simulink model "TCAF_WHOLESIM"  (R2022a)
settings: Solver=ode4  StartTime=0.0  StopTime=150  FixedStep=0.01  RelTol=1e-3  EnableMultiTasking=on
PreLoadFcn:
  | listing = dir;
  | if (contains([listing .name], 'TPF')) && (contains([listing .name], 'MAP'))
  |     addpath('./TCAF', './TRN', './FTG', './DYN', './FLCC', './GPS', './RALT', './INS', './MAP');
  | elseif (contains([listing .name], 'TCAF_WHOLESIM.slx'))
  |     addpath('./TCAF', './TRN', './FTG', '../DYN', '../FLCC', '../GPS', '../RALT', '../INS', '../MAP');
  | else
  | 
  | end
  | addpath('C:\Users\ASCL\Documents\GitHub\DTNS\MAP\MAP_DB');
  | 
  | load('BUS_STRUCTURE_DYN.mat');
  | load('BUS_STRUCTURE_FLCC.mat');
  | load('BUS_STRUCTURE_RALT.mat');
  | load('BUS_STRUCTURE_INS.mat');
  | load('BUS_STRUCTURE_GPS.mat');
  | load('BusStructureTRN.mat');
  | load('BusStructureWTPG.mat');
  | load('BusStructureDTF.mat');
  | load('BusStructureGCAWS.mat');
  | FTG_initState;
InitFcn:
  | listing = dir;
  | if (contains([listing .name], 'TPF')) && (contains([listing .name], 'MAP'))
  |     addpath('./TCAF', './TRN', './FTG', './DYN', './FLCC', './GPS', './RALT', './INS', './MAP');
  | elseif (contains([listing .name], 'TCAF_WHOLESIM.slx'))
  |     addpath('./TCAF', './TRN', './FTG', '../DYN', '../FLCC', '../GPS', '../RALT', '../INS', '../MAP');
  | else
  | 
  | end
  | 
  | load('BUS_STRUCTURE_DYN.mat');
  | load('BUS_STRUCTURE_FLCC.mat');
  | load('BUS_STRUCTURE_RALT.mat');
  | load('BUS_STRUCTURE_INS.mat');
  | load('BUS_STRUCTURE_GPS.mat');
  | load('BusStructureTRN.mat');
  | load('BusStructureWTPG.mat');
  | load('BusStructureDTF.mat');
  | load('BusStructureGCAWS.mat');
  | FTG_initState;
  | 
  | clear 'logsout'
libraries: aerolibconvert2 x14, simulink_extras x5
(part 1 of 2)
settings Model: PacingRate=3  Creator=ASCL  LastModifiedBy=ASCL
settings SolverCC: PositivePriorityOrder=on  AutoInsertRateTranBlk=on
settings DataIOCC: ExternalInput=FTGScenario.getElement('IN_STICK'), [], [], FTGScenario.getElement('IN_FLIGHT_CMD'), []  LoadExternalInput=on  SaveOutput=off  DSMLogging=off  ReturnWorkspaceOutputs=off
settings OptimizationCC: BlockReduction=off  DefaultParameterBehavior=Inlined  UseDivisionForNetSlopeComputation=on  GainParamInheritBuiltInType=on  UseFloatMulNetSlope=on  ExpressionFolding=off  PassReuseOutputArgsAs=Individual arguments  ZeroExternalMemoryAtStartup=off  ZeroInternalMemoryAtStartup=off  EfficientFloat2IntCast=on  LifeSpan=inf  OptimizeBlockOrder=speed  DifferentSizesBufferReuse=on  EfficientTunableParamExpr=on
settings DebuggingCC: SignalInfNanChecking=warning  ReadBeforeWriteMsg=EnableAllAsError  WriteAfterWriteMsg=EnableAllAsError  WriteAfterReadMsg=EnableAllAsError  IntegerOverflowMsg=error  ParameterTunabilityLossMsg=error  UniqueDataStoreMsg=error  AssertControl=DisableAll  NonBusSignalsTreatedAsBus=error  SFInvalidInputDataAccessInChartInitDiag=error  SFTransitionOutsideNaturalParentDiag=error  SFUnreachableExecutionPathDiag=error  SFUndirectedBroadcastEventsDiag=error  IntegerSaturationMsg=error
settings HardwareCC: ProdBitPerPointer=32  ProdBitPerSizeT=32  ProdBitPerPtrDiffT=32  ProdLargestAtomicInteger=Long  ProdLargestAtomicFloat=Double  ProdEndianess=BigEndian  ProdWordSize=32  ProdLongLongMode=on  ProdHWDeviceType=Freescale->MPC83xx
settings ModelReferenceCC: ModelReferenceNumInstancesAllowed=Single
settings SFSimCC: SimCustomHeaderCode="#include \"MAP.h\""  SimUserSources=MAP.c  SimUserLibraries=WS2_32.LIB  CompileTimeRecursionLimit=0  EnableRuntimeRecursion=off  MATLABDynamicMemAlloc=off  CustomCodeGlobalsAsFunctionIO=on
settings RTWCC: SystemTargetFile=ert.tlc  TemplateMakefile=ert_default_tmf  GenerateReport=on  RTWUseSimCustomCode=on  CustomHeaderCode="#include \"MAP.h\""  CustomSource=MAP.c  CustomLibrary=WS2_32.LIB  BuildConfiguration=Faster Runs  IncludeHyperlinkInReport=on  LaunchReport=on  GenerateTraceInfo=on  GenerateTraceReport=on  GenerateTraceReportSl=on  GenerateTraceReportSf=on  GenerateTraceReportEml=on
settings CodeAppCC: ForceParamTrailComments=on  IgnoreCustomStorageClasses=off  OperatorAnnotations=on  SimulinkDataObjDesc=on  SFDataObjDesc=on  MATLABFcnDesc=on  InsertBlockDesc=on  StateflowObjectComments=on  MATLABSourceComments=on  EnableCustomComments=on  InlinedPrmAccess=Macros  ReqsInCode=on
settings ERTTargetCC: TargetLangStandard=C99 (ISO)  UtilityFuncGeneration=Shared location  GenerateSampleERTMain=on  IncludeMdlTerminateFcn=off  CombineSignalStateStructs=on  SuppressErrorStatus=on  SupportAbsoluteTime=off  SupportNonFinite=off  SupportComplex=off  ParenthesesLevel=Standards  CastingMode=Standards  GenerateSharedConstants=off  InlinedParameterPlacement=NonHierarchical  ERTCustomFileTemplate=example_file_process.tlc  RateTransitionBlockCode=Function  PreserveIfCondition=on  ConvertIfToSwitch=off  EnableSignedLeftShifts=off  EnableSignedRightShifts=off

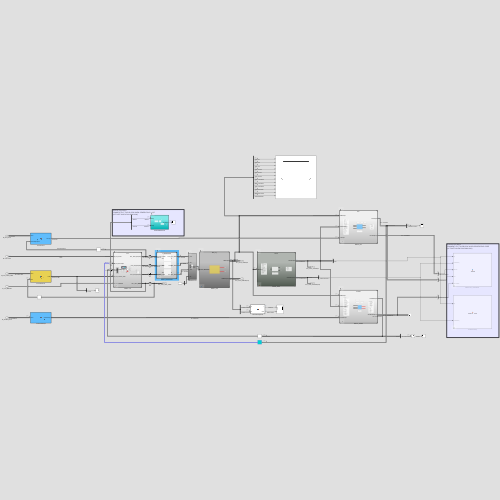
[thumbnail: Simulink's stored preview of the top-level diagram]
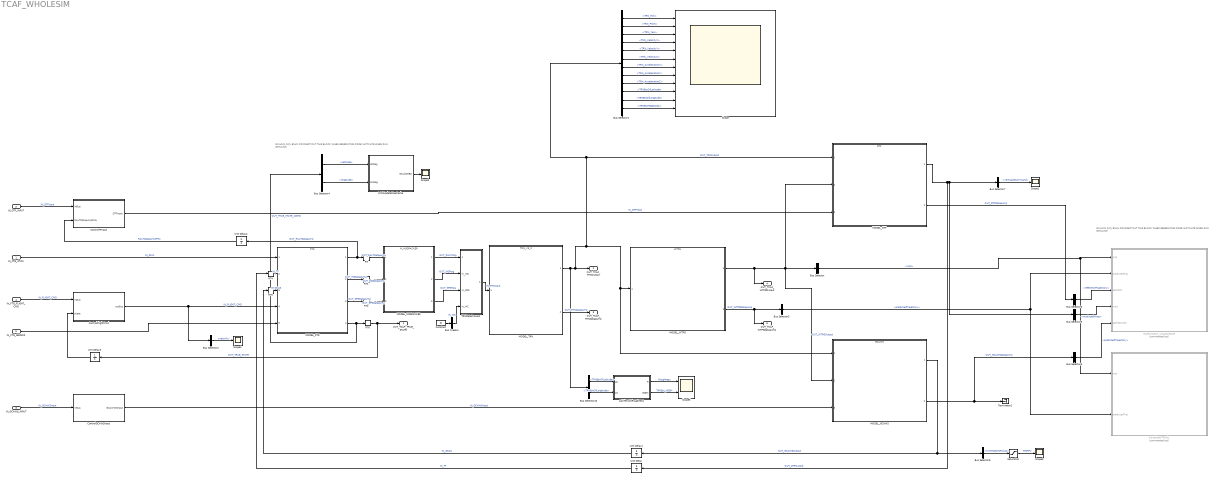
== system TCAF_WHOLESIM ==
  note: Simulink Only Block
      | COMMENT OUT THIS BLOCK WHEN GENERATING CODE
      | (ACTIVATE WHEN RUN SIMULINK)
  note: Simulink Only Block
      | COMMENT OUT THIS BLOCK WHEN GENERATING CODE
      | (ACTIVATE WHEN RUN SIMULINK)
  IN_FTG_STICK : Inport  OutDataTypeStr=Bus: BUS_FLCC_STICK  BusOutputAsStruct=on
  IN_DTF_INPUT : Inport  Port=2  OutDataTypeStr=Bus: DTFInput  BusOutputAsStruct=on
  IN_GCAWS_INPUT : Inport  Port=3  OutDataTypeStr=Bus: GCAWSInput  BusOutputAsStruct=on
  IN_FTG_FLIGHT_CMD : Inport  Port=4  OutDataTypeStr=Bus: BUS_FLCC_FLIGHT_CMD  Interpolate=off  BusOutputAsStruct=on
  IN_FTG_SENSOR : Inport  Port=5  OutDataTypeStr=Bus: BUS_SENSOR_ALL_INPUTSTATUS  BusOutputAsStruct=on
  Bus Creator : BusCreator  Inputs=1  OutDataTypeStr=Bus: TRN_MC  NonVirtualBus=on
      settings: InheritFromInputs=off
  Bus Selector : BusSelector  OutputSignals=wtp
  Bus Selector1 : BusSelector  OutputSignals=TRN_Roll,TRN_Pitch,TRN_Yaw,TRN_VelocityX,TRN_VelocityY,TRN_VelocityZ,TRN_AccelerationX,TRN_AccelerationY,TRN_AccelerationZ,TRNEstOfLatitude,TRNEstOfLongitude,TRNEstHeightAGL
  Bus Selector10 : BusSelector  OutputSignals=TRNEstOfLatitude,TRNEstOfLongitude
  Bus Selector2 : BusSelector  OutputSignals=nextAlt
  Bus Selector3 : BusSelector  OutputSignals=predictedTrajectory
  Bus Selector4 : BusSelector  OutputSignals=latitude,longitude
  Bus Selector5 : BusSelector  OutputSignals=predictedTrajectory
  Bus Selector6 : BusSelector  OutputSignals=referenceTrajectory
  Bus Selector7 : BusSelector  OutputSignals=verticalGCommand
  Bus Selector8 : BusSelector  OutputSignals=timeToGoToPullUp
  Bus Selector9 : BusSelector  OutputSignals=msdUsedWrap
  Constant : Constant  Value=0  OutDataTypeStr=boolean
  ControlFlightCmd : MATLAB Function  TreatAsAtomicUnit=on
  ControlGCAWSInput : MATLAB Function  TreatAsAtomicUnit=on
  ControlTFInput : MATLAB Function  TreatAsAtomicUnit=on
  InitNUpdateMapCache : Subsystem  TreatAsAtomicUnit=on  ScheduleAs=Periodic partition  PartitionName=InitNUpdateMapCache  SystemSampleTime=0.01
  MATFunction_VisualizeWCP : MATLAB Function  Commented=on  TreatAsAtomicUnit=on
  MODEL_DTF : ModelReference  ModelNameDialog=DTF.slx  SimulationMode=Normal  ScheduleRates=on  ScheduleRatesWith=Schedule Editor  ModelReferenceVersion=1.433
  MODEL_FTG : ModelReference  ModelNameDialog=FTG.slx  SimulationMode=Normal  ScheduleRates=on  ScheduleRatesWith=Schedule Editor  ModelReferenceVersion=1.514
  MODEL_GCAWS : ModelReference  ModelNameDialog=GCAWS.slx  SimulationMode=Normal  ScheduleRates=on  ScheduleRatesWith=Schedule Editor  ModelReferenceVersion=1.778
  MODEL_MSGPACKER : ModelReference  ModelNameDialog=M_MSGPACKER.slx  SimulationMode=Normal  ScheduleRates=on  ScheduleRatesWith=Schedule Editor  ModelReferenceVersion=1.311
  MODEL_TRN : ModelReference  ModelNameDialog=TRN_V3_2.slx  SimulationMode=Normal  ScheduleRates=on  ScheduleRatesWith=Schedule Editor  CachedPortDiscreteRates=[0.04]  ModelReferenceVersion=2.345
  MODEL_WTPG : ModelReference  ModelNameDialog=WTPG.slx  SimulationMode=Normal  ScheduleRates=on  ScheduleRatesWith=Schedule Editor  ModelReferenceVersion=1.378
  RT{,1..2,4..5} (5 alike) : RateTransition
  RT6 : RateTransition  OutPortSampleTime=0.04
  Saturation : Saturate  UpperLimit=5.0  LowerLimit=0.0
  Scope : Scope  NumInputPorts=12
  Scope{1..4} (4 alike) : Scope
  Scope5 : Scope  NumInputPorts=2
  TRNDataProcess : Subsystem  TreatAsAtomicUnit=on  ScheduleAs=Periodic partition  PartitionName=TRNDataProcess  SystemSampleTime=0.04
  Terminator2 : Terminator
  Unit Delay{,1..3} (4 alike) : UnitDelay  SampleTime=-1  HasFrameUpgradeWarning=on
  VisualizeWTPOnly : MATLAB Function  Commented=on  TreatAsAtomicUnit=on
  calcTerrainRoughness : MATLAB Function  TreatAsAtomicUnit=on
  OUT_TCAF_TRUE_STATE : Outport  OutDataTypeStr=Bus: BUS_DYN_STATE  BusOutputAsStruct=on
  OUT_TCAF_TRNOutput : Outport  Port=2  OutDataTypeStr=Bus: TRNOutput  BusOutputAsStruct=on
  OUT_TCAF_TRNDatapump : Outport  Port=3  OutDataTypeStr=Bus: TRNDatapump
  OUT_TCAF_WTPGOutput : Outport  Port=4  OutDataTypeStr=Bus: WTPGOutput
  OUT_TCAF_WTPGDatapump : Outport  Port=5  OutDataTypeStr=Bus: WTPGDatapump
  wires:
  Bus Selector7/1 -> Scope1/1  "<verticalGCommand>"
  Bus Selector6/1 -> MATFunction_VisualizeWCP/3(pathDTF)  "<referenceTrajectory>"
  Bus Selector1/4 -> Scope/4  "<TRN_VelocityX>"
  MODEL_DTF/2 -> Bus Selector6/1  "OUT_DTFDatapump"
  Bus Creator/1 -> TRNDataProcess/4(In_MC)  "IN_MC"
  Bus Selector5/1 -> MATFunction_VisualizeWCP/5(pathGCAWS)  "<predictedTrajectory>"
  Bus Selector1/5 -> Scope/5  "<TRN_VelocityY>"
  Bus Selector1/7 -> Scope/7  "<TRN_AccelerationX>"
  Bus Selector1/8 -> Scope/8  "<TRN_AccelerationY>"
  MODEL_WTPG/1 -> OUT_TCAF_WTPGOutput/1, MODEL_GCAWS/2, MODEL_DTF/2, Bus Selector/1  "OUT_WTPGOutput"
  Bus Selector1/9 -> Scope/9  "<TRN_AccelerationZ>"
  Bus Selector1/12 -> Scope/12  "<TRNEstHeightAGL>"
  Bus Selector1/11 -> Scope/11  "<TRNEstOfLongitude>"
  MODEL_FTG/3 -> RT2/1  "OUT_GPSDatapump"
  MODEL_WTPG/2 -> OUT_TCAF_WTPGDatapump/1, Bus Selector3/1  "OUT_WTPGDatapump"
  Bus Selector1/3 -> Scope/3  "<TRN_Yaw>"
  MODEL_GCAWS/2 -> Bus Selector5/1, Terminator2/1  "OUT_GCAWSDatapump"
  Bus Selector1/10 -> Scope/10  "<TRNEstOfLatitude>"
  MODEL_TRN/2 -> OUT_TCAF_TRNDatapump/1  "OUT_TRNDatapump"
  MODEL_GCAWS/1 -> Unit Delay1/1, Bus Selector8/1  "OUT_GCAWSOutput"
  Bus Selector1/6 -> Scope/6  "<TRN_VelocityZ>"
  Bus Selector3/1 -> VisualizeWTPOnly/2(predictedTraj), MATFunction_VisualizeWCP/2(predictedTraj)  "<predictedTrajectory>"
  Constant/1 -> Bus Creator/1
  IN_GCAWS_INPUT/1 -> ControlGCAWSInput/1(inBus)  "IN_GCAWSInput"
  IN_FTG_FLIGHT_CMD/1 -> ControlFlightCmd/1(inBus)  "IN_FLIGHT_CMD"
  RT6/1 -> Unit Delay3/1, OUT_TCAF_TRUE_STATE/1  "OUT_TRUE_STATE"
  Bus Selector4/2 -> InitNUpdateMapCache/2(lonDeg)  "<longitude>"
  MODEL_FTG/2 -> RT1/1  "OUT_INSDatapump"
  Unit Delay1/1 -> RT5/1  "IN_GCAS"
  Unit Delay/1 -> RT4/1  "IN_TF"
  MODEL_FTG/1 -> RT/1, Unit Delay2/1  "OUT_RALTDatapump"
  Bus Selector/1 -> VisualizeWTPOnly/1(wtp), MATFunction_VisualizeWCP/1(wtp)  "<wtp>"
  Bus Selector1/1 -> Scope/1  "<TRN_Roll>"
  IN_FTG_STICK/1 -> MODEL_FTG/1  "IN_Stick"
  MODEL_DTF/1 -> Bus Selector9/1, Bus Selector7/1, Unit Delay/1  "OUT_DTFOutput"
  Bus Selector1/2 -> Scope/2  "<TRN_Pitch>"
  Bus Selector8/1 -> Saturation/1  "<timeToGoToPullUp>"
  Saturation/1 -> Scope3/1  "TTGTPU"
  ControlFlightCmd/1(outBus) -> Bus Selector2/1, MODEL_FTG/4  "IN_FLIGHT_CMD"
  IN_DTF_INPUT/1 -> ControlTFInput/1(inBus)  "IN_DTFInput"
  MODEL_MSGPACKER/3 -> TRNDataProcess/3(In_GPS)  "OUT_GPSMsg"
  MODEL_MSGPACKER/1 -> TRNDataProcess/1(In_RALT)  "OUT_RALTMsg"
  MODEL_MSGPACKER/2 -> TRNDataProcess/2(In_INS)  "OUT_INSMsg"
  InitNUpdateMapCache/1(resultDTED) -> Scope2/1
  IN_FTG_SENSOR/1 -> MODEL_FTG/5
  ControlTFInput/1(DTFInput) -> MODEL_DTF/3  "IN_DTFInput"
  Unit Delay2/1 -> ControlTFInput/2(RALTDatapumpPrev)  "RALTDatapumpPrev"
  Bus Selector2/1 -> Scope4/1  "<nextAlt>"
  ControlGCAWSInput/1(GCAWWSInput) -> MODEL_GCAWS/3  "IN_GCAWSInput"
  Bus Selector9/1 -> MATFunction_VisualizeWCP/4(msd)  "<msdUsedWrap>"
  Unit Delay3/1 -> ControlFlightCmd/2(state)
  TRNDataProcess/1(TRN INPUT) -> MODEL_TRN/1  "IN_TRNInput"
  RT/1 -> MODEL_MSGPACKER/1  "OUT_RALTDatapump"
  RT1/1 -> MODEL_MSGPACKER/2  "OUT_INSDatapump"
  RT2/1 -> MODEL_MSGPACKER/3  "OUT_GPSDatapump"
  Bus Selector4/1 -> InitNUpdateMapCache/1(latDeg)  "<latitude>"
  RT4/1 -> MODEL_FTG/2  "IN_TF"
  RT5/1 -> MODEL_FTG/3  "IN_GCAS"
  MODEL_FTG/4 -> Bus Selector4/1, RT6/1  "OUT_TRUE_STATE_100HZ"
  MODEL_TRN/1 -> MODEL_GCAWS/1, MODEL_WTPG/1, Bus Selector1/1, MODEL_DTF/1, OUT_TCAF_TRNOutput/1, Bus Selector10/1  "OUT_TRNOutput"
  calcTerrainRoughness/1(R) -> Scope5/1  "Roughness"
  calcTerrainRoughness/2(hDEM) -> Scope5/2  "TRNEst_hDEM"
  Bus Selector10/2 -> calcTerrainRoughness/2(lon)  "<TRNEstOfLongitude>"
  Bus Selector10/1 -> calcTerrainRoughness/1(lat)  "<TRNEstOfLatitude>"

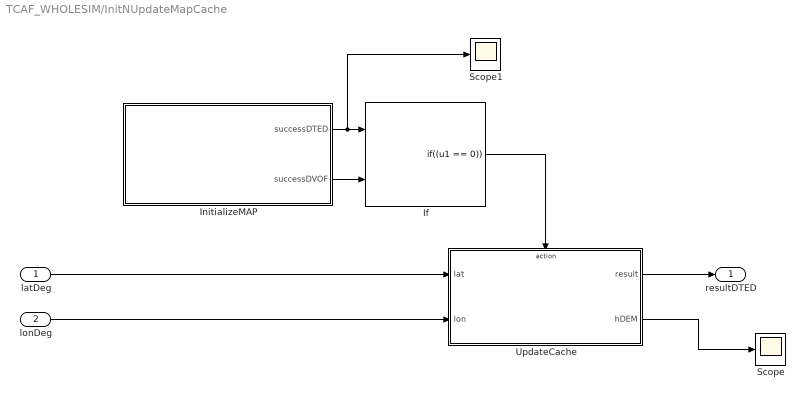
== system TCAF_WHOLESIM/InitNUpdateMapCache ==
  latDeg : Inport  OutDataTypeStr=double
  lonDeg : Inport  Port=2  OutDataTypeStr=double
  If : If  NumInputs=2  IfExpression=(u1 == 0)  ShowElse=off
  InitializeMAP : MATLAB Function  TreatAsAtomicUnit=on
  Scope : Scope
  Scope1 : Scope
  UpdateCache : Subsystem  TreatAsAtomicUnit=on
  resultDTED : Outport  VectorParamsAs1DForOutWhenUnconnected=off
  wires:
  lonDeg/1 -> UpdateCache/2(lon)
  UpdateCache/1(result) -> resultDTED/1
  InitializeMAP/1(successDTED) -> Scope1/1, If/1
  latDeg/1 -> UpdateCache/1(lat)
  InitializeMAP/2(successDVOF) -> If/2
  If/1 -> UpdateCache/Action
  UpdateCache/2(hDEM) -> Scope/1

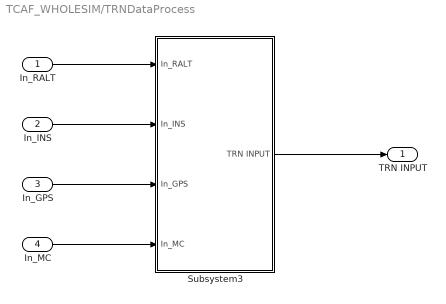
== system TCAF_WHOLESIM/TRNDataProcess ==
  In_RALT : Inport
  In_INS : Inport  Port=2
  In_GPS : Inport  Port=3
  In_MC : Inport  Port=4
  Subsystem3 : Subsystem
  TRN INPUT : Outport
  wires:
  In_GPS/1 -> Subsystem3/3(In_GPS)
  In_MC/1 -> Subsystem3/4(In_MC)
  Subsystem3/1(TRN INPUT) -> TRN INPUT/1
  In_RALT/1 -> Subsystem3/1(In_RALT)
  In_INS/1 -> Subsystem3/2(In_INS)

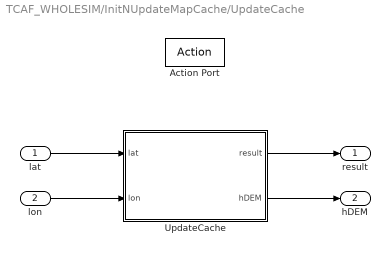
== system TCAF_WHOLESIM/InitNUpdateMapCache/UpdateCache ==
  lat : Inport
  lon : Inport  Port=2
  Action Port : ActionPort  ActionPortLabel=if((u1 == 0))
  UpdateCache : MATLAB Function  TreatAsAtomicUnit=on
  result : Outport  VectorParamsAs1DForOutWhenUnconnected=off
  hDEM : Outport  Port=2
  wires:
  UpdateCache/1(result) -> result/1
  lat/1 -> UpdateCache/1(lat)
  lon/1 -> UpdateCache/2(lon)
  UpdateCache/2(hDEM) -> hDEM/1

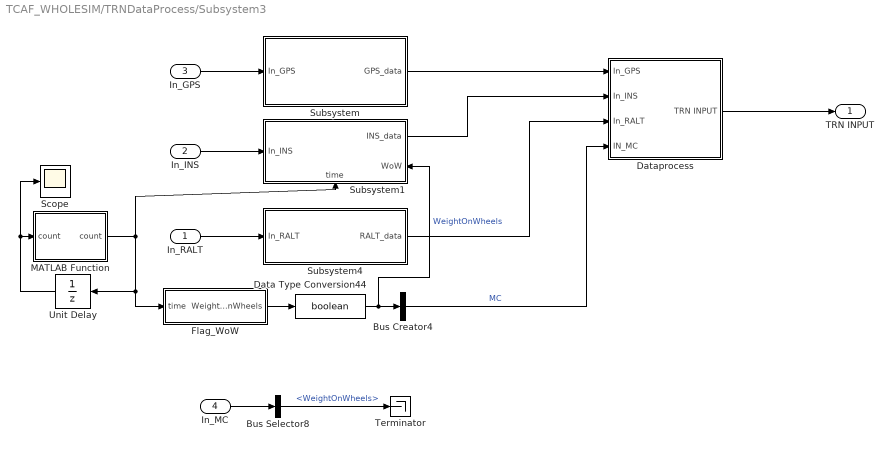
== system TCAF_WHOLESIM/TRNDataProcess/Subsystem3 ==
  In_RALT : Inport
  In_INS : Inport  Port=2
  In_GPS : Inport  Port=3
  In_MC : Inport  Port=4
  Bus Creator4 : BusCreator  Inputs=1  OutDataTypeStr=Bus: TRN_MC
  Bus Selector8 : BusSelector  OutputSignals=WeightOnWheels
  Data Type Conversion44 : DataTypeConversion  OutDataTypeStr=boolean  SaturateOnIntegerOverflow=off  RndMeth=Floor
  Dataprocess : Subsystem
  Flag_WoW : MATLAB Function  TreatAsAtomicUnit=on
  MATLAB Function : MATLAB Function  TreatAsAtomicUnit=on
  Scope : Scope
  Subsystem : Subsystem
  Subsystem1 : Subsystem
      settings: PortSchema="{\"entries\":[{\"content\":{\"sides\":[{\"content\":{\"connectorIds\":[\"In1\"]},\"type\":\"ConnectorPlacement.EquallySpacedRectSide\",\"uuid\":\"627687e9-0c69-45fe-ab30-f2b8c78c94c9\"},{\"content\":{\"connectorIds\":[\"Out1\",\"In3\"],\"side\":\"RIGHT\"},\"type\":\"ConnectorPlacement.EquallySpacedRectSide\",\"uuid\":\"cca5eff4-b683-4134-86dd-9b38fc1aef42\"},{\"content\":{\"connectorIds\":[],\"side\":\"TOP\"},\"type\":\"ConnectorPlacement.EquallySpacedRectSide\",\"uuid\":\"db09404b-1405-40a7-9047-09d57f6d1ee9\"},{\"content\":{\"connectorIds\":[\"In2\"],\"side\":\"BOTTOM\"},\"type\":\"ConnectorPlacement.EquallySpacedRectSide\",\"uuid\":\"43181e0c-7a64-4398-bddd-a3419aca840e\"}]},\"type\":\"ConnectorPlacement.EquallySpacedConnector\",\"uuid\":\"8e5a566a-2f6b-4dcc-950b-8518900682ca\"}],\"packageUris\":[\"http://schema.mathworks.com/mf0/Connector/R2020b\"],\"version\":\"1.0\"}"
  Subsystem4 : Subsystem
  Terminator : Terminator
  Unit Delay : UnitDelay  SampleTime=-1  HasFrameUpgradeWarning=on
  TRN INPUT : Outport
  wires:
  Flag_WoW/1(WeightOnWheels) -> Data Type Conversion44/1
  Data Type Conversion44/1 -> Subsystem1/3(WoW), Bus Creator4/1  "WeightOnWheels"
  Subsystem1/1(INS_data) -> Dataprocess/2(In_INS)
  Bus Creator4/1 -> Dataprocess/4(IN_MC)  "MC"
  Subsystem/1(GPS_data) -> Dataprocess/1(In_GPS)
  Dataprocess/1(TRN INPUT) -> TRN INPUT/1
  In_MC/1 -> Bus Selector8/1
  In_GPS/1 -> Subsystem/1(In_GPS)
  In_INS/1 -> Subsystem1/1(In_INS)
  In_RALT/1 -> Subsystem4/1(In_RALT)
  Subsystem4/1(RALT_data) -> Dataprocess/3(In_RALT)
  MATLAB Function/1(count) -> Unit Delay/1, Flag_WoW/1(time), Subsystem1/2(time)
  Unit Delay/1 -> Scope/1, MATLAB Function/1("count ")
  Bus Selector8/1 -> Terminator/1  "<WeightOnWheels>"

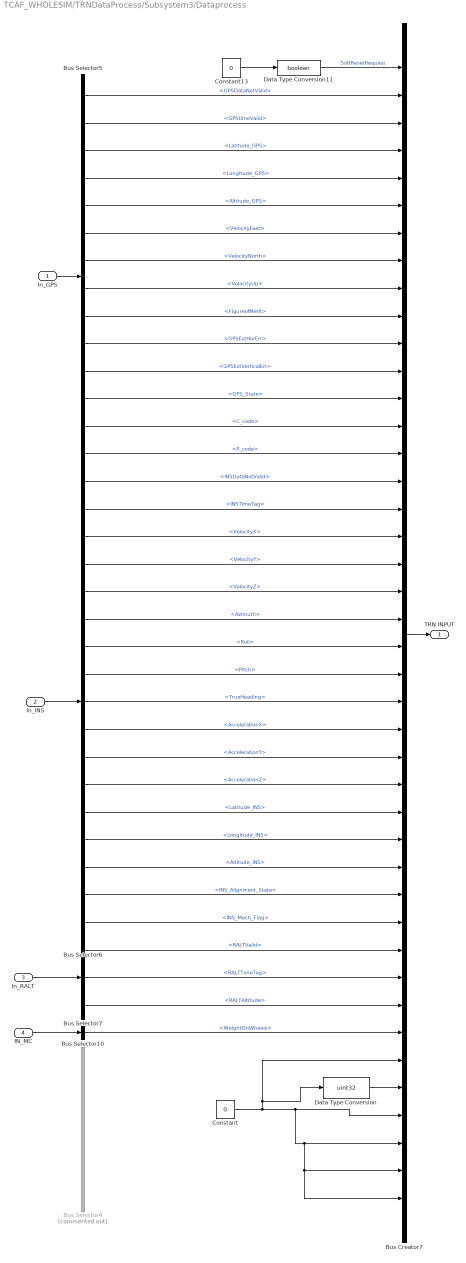
== system TCAF_WHOLESIM/TRNDataProcess/Subsystem3/Dataprocess ==
  In_GPS : Inport
  In_INS : Inport  Port=2
  In_RALT : Inport  Port=3
  IN_MC : Inport  Port=4
  Bus Creator7 : BusCreator  Inputs=42  OutDataTypeStr=Bus: TRNInput
  Bus Selector10 : BusSelector  OutputSignals=WeightOnWheels
  Bus Selector4 : BusSelector  Commented=on  OutputSignals=MAP_hight,Map_Level,Map_size,Map_resolution,bottomLat,leftLon
  Bus Selector5 : BusSelector  OutputSignals=GPSDataNotValid,GPStimeValid,Latitude_GPS,Longitude_GPS,Altitude_GPS,VelocityEast,VelocityNorth,VelocityUp,FigureofMerit,GPSEstHorErr,GPSEstVerticalErr,GPS_State,C_code,P_code
  Bus Selector6 : BusSelector  OutputSignals=INSDataNotValid,INSTimeTag,VelocityX,VelocityY,VelocityZ,Azimuth,Roll,Pitch,TrueHeading,AccelerationX,AccelerationY,AccelerationZ,Latitude_INS,Longitude_INS,Altitude_INS,INS_Alignment_State,INS_Mech_Flag
  Bus Selector7 : BusSelector  OutputSignals=RALTValid,RALTTimeTag,RALTAltitude
  Constant : Constant  Value=0
  Constant13 : Constant  Value=0
  Data Type Conversion : DataTypeConversion  OutDataTypeStr=uint32  SaturateOnIntegerOverflow=off  RndMeth=Floor
  Data Type Conversion11 : DataTypeConversion  OutDataTypeStr=boolean  SaturateOnIntegerOverflow=off  RndMeth=Floor
  TRN INPUT : Outport  OutDataTypeStr=Bus: TRNInput  VectorParamsAs1DForOutWhenUnconnected=off
  wires:
  Bus Selector5/8 -> Bus Creator7/9  "<VelocityUp>"
  Bus Selector6/16 -> Bus Creator7/31  "<INS_Alignment_State>"
  Bus Selector5/7 -> Bus Creator7/8  "<VelocityNorth>"
  In_GPS/1 -> Bus Selector5/1
  Bus Selector5/4 -> Bus Creator7/5  "<Longitude_GPS>"
  Bus Selector5/11 -> Bus Creator7/12  "<GPSEstVerticalErr>"
  Bus Selector5/3 -> Bus Creator7/4  "<Latitude_GPS>"
  Bus Selector6/13 -> Bus Creator7/28  "<Latitude_INS>"
  Bus Selector6/14 -> Bus Creator7/29  "<Longitude_INS>"
  Bus Selector5/12 -> Bus Creator7/13  "<GPS_State>"
  Bus Selector6/9 -> Bus Creator7/24  "<TrueHeading>"
  Bus Selector5/14 -> Bus Creator7/15  "<P_code>"
  Bus Selector6/1 -> Bus Creator7/16  "<INSDataNotValid>"
  Bus Creator7/1 -> TRN INPUT/1
  Data Type Conversion11/1 -> Bus Creator7/1  "SoftResetRequest"
  Bus Selector5/6 -> Bus Creator7/7  "<VelocityEast>"
  Bus Selector6/12 -> Bus Creator7/27  "<AccelerationZ>"
  Bus Selector6/3 -> Bus Creator7/18  "<VelocityX>"
  Bus Selector5/13 -> Bus Creator7/14  "<C_code>"
  Bus Selector6/6 -> Bus Creator7/21  "<Azimuth>"
  Bus Selector5/5 -> Bus Creator7/6  "<Altitude_GPS>"
  Bus Selector6/10 -> Bus Creator7/25  "<AccelerationX>"
  Bus Selector7/3 -> Bus Creator7/35  "<RALTAltitude>"
  In_INS/1 -> Bus Selector6/1
  Bus Selector7/1 -> Bus Creator7/33  "<RALTValid>"
  Bus Selector5/1 -> Bus Creator7/2  "<GPSDataNotValid>"
  Bus Selector10/1 -> Bus Creator7/36  "<WeightOnWheels>"
  Bus Selector6/17 -> Bus Creator7/32  "<INS_Mech_Flag>"
  Bus Selector6/4 -> Bus Creator7/19  "<VelocityY>"
  Bus Selector6/7 -> Bus Creator7/22  "<Roll>"
  Constant13/1 -> Data Type Conversion11/1
  Bus Selector7/2 -> Bus Creator7/34  "<RALTTimeTag>"
  Bus Selector6/5 -> Bus Creator7/20  "<VelocityZ>"
  Bus Selector6/2 -> Bus Creator7/17  "<INSTimeTag>"
  Bus Selector6/8 -> Bus Creator7/23  "<Pitch>"
  Bus Selector5/2 -> Bus Creator7/3  "<GPStimeValid>"
  Bus Selector5/10 -> Bus Creator7/11  "<GPSEstHorErr>"
  Bus Selector6/15 -> Bus Creator7/30  "<Altitude_INS>"
  Bus Selector6/11 -> Bus Creator7/26  "<AccelerationY>"
  Bus Selector5/9 -> Bus Creator7/10  "<FigureofMerit>"
  In_RALT/1 -> Bus Selector7/1
  IN_MC/1 -> Bus Selector10/1
  Constant/1 -> Bus Creator7/39, Bus Creator7/40, Bus Creator7/42, Bus Creator7/41, Bus Creator7/37, Data Type Conversion/1
  Data Type Conversion/1 -> Bus Creator7/38

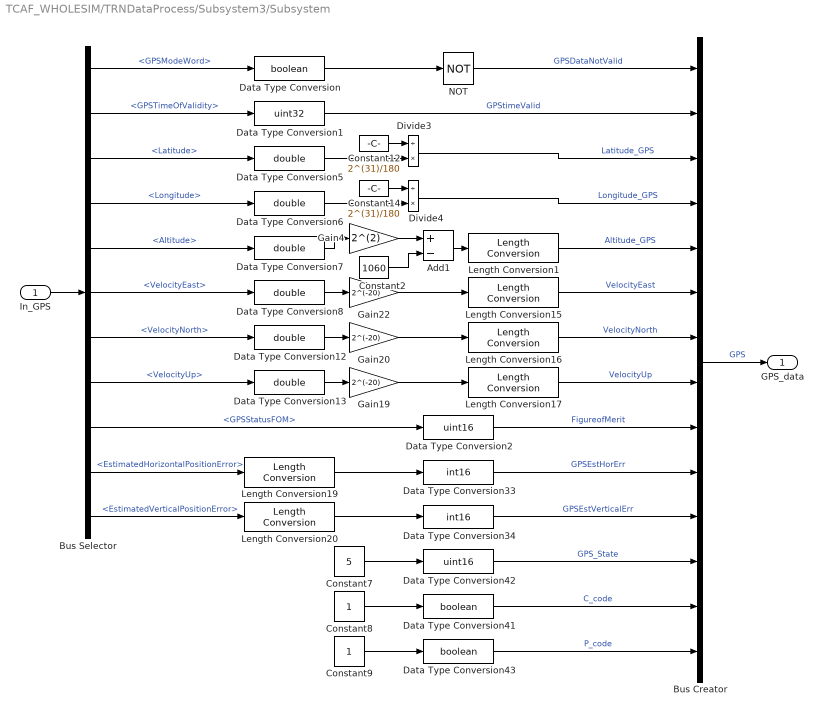
== system TCAF_WHOLESIM/TRNDataProcess/Subsystem3/Subsystem ==
  In_GPS : Inport
  Add1 : Sum  Inputs=+-
  Bus Creator : BusCreator  Inputs=14  OutDataTypeStr=Bus: TRN_GPS
  Bus Selector : BusSelector  OutputSignals=GPSModeWord,GPSTimeOfValidity,Latitude,Longitude,Altitude,VelocityEast,VelocityNorth,VelocityUp,GPSStatusFOM,EstimatedHorizontalPositionError,EstimatedVerticalPositionError
  Constant12 : Constant  Value=2^(31)/180
  Constant14 : Constant  Value=2^(31)/180
  Constant2 : Constant  Value=1060
  Constant7 : Constant  Value=5
  Constant8 : Constant
  Constant9 : Constant
  Data Type Conversion : DataTypeConversion  OutDataTypeStr=boolean  SaturateOnIntegerOverflow=off  RndMeth=Floor
  Data Type Conversion1 : DataTypeConversion  OutDataTypeStr=uint32  SaturateOnIntegerOverflow=off  RndMeth=Floor
  Data Type Conversion{5..8,12..13} (6 alike) : DataTypeConversion  OutDataTypeStr=double  SaturateOnIntegerOverflow=off  RndMeth=Floor
  Data Type Conversion2 : DataTypeConversion  OutDataTypeStr=uint16  SaturateOnIntegerOverflow=off  RndMeth=Floor
  Data Type Conversion33 : DataTypeConversion  OutDataTypeStr=int16  SaturateOnIntegerOverflow=off  RndMeth=Floor
  Data Type Conversion34 : DataTypeConversion  OutDataTypeStr=int16  SaturateOnIntegerOverflow=off  RndMeth=Floor
  Data Type Conversion41 : DataTypeConversion  OutDataTypeStr=boolean  SaturateOnIntegerOverflow=off  RndMeth=Floor
  Data Type Conversion42 : DataTypeConversion  OutDataTypeStr=uint16  SaturateOnIntegerOverflow=off  RndMeth=Floor
  Data Type Conversion43 : DataTypeConversion  OutDataTypeStr=boolean  SaturateOnIntegerOverflow=off  RndMeth=Floor
  Divide3 : Product  Inputs=/*
  Divide4 : Product  Inputs=/*
  Gain19 : Gain  Gain=2^(-20)
  Gain20 : Gain  Gain=2^(-20)
  Gain22 : Gain  Gain=2^(-20)
  Gain4 : Gain  Gain=2^(2)
  Length Conversion{1,15..17,19..20} (6 alike) : aerolibconvert2/Length Conversion  IU=ft  OU=m
  NOT : Logic  Operator=NOT  IconShape=distinctive  AllPortsSameDT=off  OutDataTypeStr=boolean
  GPS_data : Outport
  wires:
  Length Conversion1/1 -> Bus Creator/5  "Altitude_GPS"
  Bus Selector/7 -> Data Type Conversion12/1  "<VelocityNorth>"
  Bus Selector/2 -> Data Type Conversion1/1  "<GPSTimeOfValidity>"
  Bus Selector/3 -> Data Type Conversion5/1  "<Latitude>"
  Gain4/1 -> Add1/1
  Data Type Conversion33/1 -> Bus Creator/10  "GPSEstHorErr"
  Bus Selector/5 -> Data Type Conversion7/1  "<Altitude>"
  Data Type Conversion8/1 -> Gain22/1
  Data Type Conversion41/1 -> Bus Creator/13  "C_code"
  Bus Selector/11 -> Length Conversion20/1  "<EstimatedVerticalPositionError>"
  Gain20/1 -> Length Conversion16/1
  Bus Selector/10 -> Length Conversion19/1  "<EstimatedHorizontalPositionError>"
  Divide3/1 -> Bus Creator/3  "Latitude_GPS"
  Bus Selector/6 -> Data Type Conversion8/1  "<VelocityEast>"
  Data Type Conversion13/1 -> Gain19/1
  Data Type Conversion6/1 -> Divide4/2
  Data Type Conversion34/1 -> Bus Creator/11  "GPSEstVerticalErr"
  Data Type Conversion42/1 -> Bus Creator/12  "GPS_State"
  Gain22/1 -> Length Conversion15/1
  Length Conversion20/1 -> Data Type Conversion34/1
  Data Type Conversion5/1 -> Divide3/2
  Add1/1 -> Length Conversion1/1
  Data Type Conversion1/1 -> Bus Creator/2  "GPStimeValid"
  Gain19/1 -> Length Conversion17/1
  Constant8/1 -> Data Type Conversion41/1
  Data Type Conversion2/1 -> Bus Creator/9  "FigureofMerit"
  Data Type Conversion7/1 -> Gain4/1
  Bus Selector/8 -> Data Type Conversion13/1  "<VelocityUp>"
  Constant7/1 -> Data Type Conversion42/1
  Bus Selector/4 -> Data Type Conversion6/1  "<Longitude>"
  Bus Selector/9 -> Data Type Conversion2/1  "<GPSStatusFOM>"
  Length Conversion17/1 -> Bus Creator/8  "VelocityUp"
  Length Conversion16/1 -> Bus Creator/7  "VelocityNorth"
  Bus Creator/1 -> GPS_data/1  "GPS"
  Data Type Conversion12/1 -> Gain20/1
  Constant2/1 -> Add1/2
  Length Conversion15/1 -> Bus Creator/6  "VelocityEast"
  Length Conversion19/1 -> Data Type Conversion33/1
  Divide4/1 -> Bus Creator/4  "Longitude_GPS"
  Constant9/1 -> Data Type Conversion43/1
  In_GPS/1 -> Bus Selector/1
  Constant14/1 -> Divide4/1
  Constant12/1 -> Divide3/1
  Data Type Conversion43/1 -> Bus Creator/14  "P_code"
  Data Type Conversion/1 -> NOT/1
  Bus Selector/1 -> Data Type Conversion/1  "<GPSModeWord>"
  NOT/1 -> Bus Creator/1  "GPSDataNotValid"

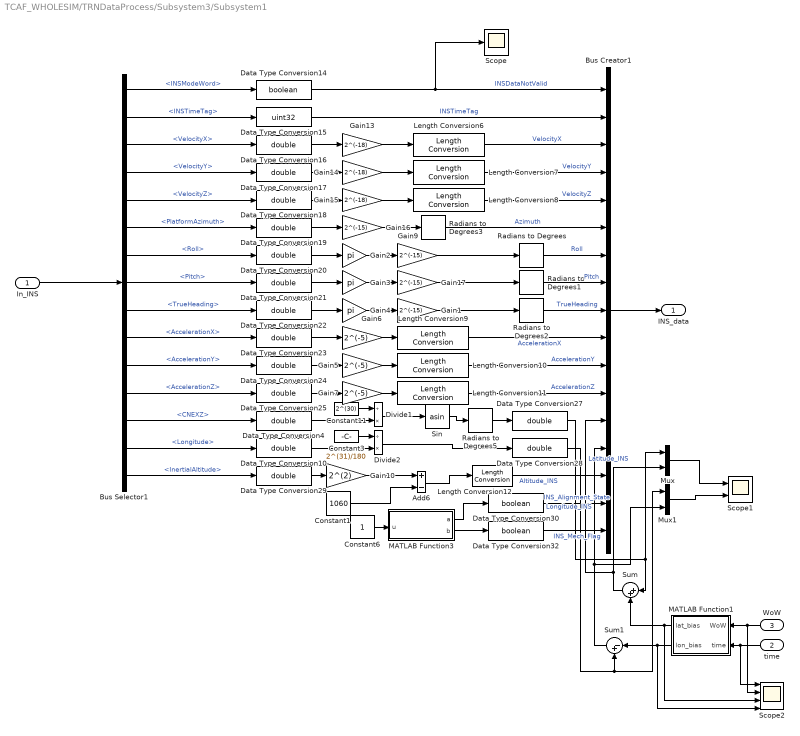
== system TCAF_WHOLESIM/TRNDataProcess/Subsystem3/Subsystem1 ==
  In_INS : Inport
  time : Inport  Port=2
  WoW : Inport  Port=3
  Add6 : Sum  Inputs=+-
  Bus Creator1 : BusCreator  Inputs=17  OutDataTypeStr=Bus: TRN_INS
  Bus Selector1 : BusSelector  OutputSignals=INSModeWord,INSTimeTag,VelocityX,VelocityY,VelocityZ,PlatformAzimuth,Roll,Pitch,TrueHeading,AccelerationX,AccelerationY,AccelerationZ,CNEXZ,Longitude,InertialAltitude
  Constant1 : Constant  Value=1060
  Constant11 : Constant  Value=2^(30)
  Constant3 : Constant  Value=2^(31)/180
  Constant6 : Constant
  Data Type Conversion{4,10,16..25,27..29} (15 alike) : DataTypeConversion  OutDataTypeStr=double  SaturateOnIntegerOverflow=off  RndMeth=Floor
  Data Type Conversion14 : DataTypeConversion  OutDataTypeStr=boolean  SaturateOnIntegerOverflow=off  RndMeth=Floor
  Data Type Conversion15 : DataTypeConversion  OutDataTypeStr=uint32  SaturateOnIntegerOverflow=off  RndMeth=Floor
  Data Type Conversion30 : DataTypeConversion  OutDataTypeStr=boolean  SaturateOnIntegerOverflow=off  RndMeth=Floor
  Data Type Conversion32 : DataTypeConversion  OutDataTypeStr=boolean  SaturateOnIntegerOverflow=off  RndMeth=Floor
  Divide1 : Product  Inputs=/*
  Divide2 : Product  Inputs=/*
  Gain{1,9,16..17} (4 alike) : Gain  Gain=2^(-15)
  Gain10 : Gain  Gain=2^(2)
  Gain13 : Gain  Gain=2^(-18)
  Gain14 : Gain  Gain=2^(-18)
  Gain15 : Gain  Gain=2^(-18)
  Gain2 : Gain  Gain=pi
  Gain3 : Gain  Gain=pi
  Gain4 : Gain  Gain=pi
  Gain5 : Gain  Gain=2^(-5)
  Gain6 : Gain  Gain=2^(-5)
  Gain7 : Gain  Gain=2^(-5)
  Length Conversion{6..12} (7 alike) : aerolibconvert2/Length Conversion  IU=ft  OU=m
  MATLAB Function1 : MATLAB Function  TreatAsAtomicUnit=on
  MATLAB Function3 : MATLAB Function  TreatAsAtomicUnit=on
  Mux : Mux  Inputs=2
  Mux1 : Mux  Inputs=2
  Radians to Degrees{,1..3,5} (5 alike) : simulink_extras/Transformations/Radians to Degrees
  Scope : Scope
  Scope1 : Scope  NumInputPorts=2
  Scope2 : Scope  NumInputPorts=4
  Sin : Trigonometry  Operator=asin
  Sum : Sum  Inputs=|++
  Sum1 : Sum  Inputs=|-+
  INS_data : Outport
  wires:
  Length Conversion6/1 -> Bus Creator1/3  "VelocityX"
  Constant6/1 -> MATLAB Function3/1(u)
  MATLAB Function3/2(b) -> Data Type Conversion32/1
  Data Type Conversion32/1 -> Bus Creator1/17  "INS_Mech_Flag"
  Data Type Conversion22/1 -> Gain4/1
  Length Conversion9/1 -> Bus Creator1/10  "AccelerationX"
  Data Type Conversion29/1 -> Gain10/1
  Radians to Degrees2/1 -> Bus Creator1/9  "TrueHeading"
  Data Type Conversion16/1 -> Gain13/1
  Data Type Conversion18/1 -> Gain15/1
  Data Type Conversion15/1 -> Bus Creator1/2  "INSTimeTag"
  Bus Selector1/14 -> Data Type Conversion10/1  "<Longitude>"
  Radians to Degrees5/1 -> Data Type Conversion27/1
  Data Type Conversion24/1 -> Gain5/1
  Sin/1 -> Radians to Degrees5/1
  Constant1/1 -> Add6/2
  Gain14/1 -> Length Conversion7/1
  Data Type Conversion14/1 -> Scope/1, Bus Creator1/1  "INSDataNotValid"
  Bus Selector1/5 -> Data Type Conversion18/1  "<VelocityZ>"
  Data Type Conversion25/1 -> Gain7/1
  Divide2/1 -> Data Type Conversion28/1
  MATLAB Function3/1(a) -> Data Type Conversion30/1
  Data Type Conversion19/1 -> Gain16/1
  Bus Selector1/10 -> Data Type Conversion23/1  "<AccelerationX>"
  Data Type Conversion20/1 -> Gain2/1
  Bus Selector1/6 -> Data Type Conversion19/1  "<PlatformAzimuth>"
  Data Type Conversion23/1 -> Gain6/1
  Bus Selector1/7 -> Data Type Conversion20/1  "<Roll>"
  Bus Selector1/2 -> Data Type Conversion15/1  "<INSTimeTag>"
  Bus Selector1/4 -> Data Type Conversion17/1  "<VelocityY>"
  Bus Selector1/3 -> Data Type Conversion16/1  "<VelocityX>"
  Add6/1 -> Length Conversion12/1
  Bus Selector1/15 -> Data Type Conversion29/1  "<InertialAltitude>"
  Bus Selector1/12 -> Data Type Conversion25/1  "<AccelerationZ>"
  Bus Selector1/13 -> Data Type Conversion4/1  "<CNEXZ>"
  Data Type Conversion4/1 -> Divide1/2
  Bus Selector1/9 -> Data Type Conversion22/1  "<TrueHeading>"
  Gain15/1 -> Length Conversion8/1
  Bus Selector1/11 -> Data Type Conversion24/1  "<AccelerationY>"
  Length Conversion12/1 -> Bus Creator1/15  "Altitude_INS"
  Gain6/1 -> Length Conversion9/1
  Data Type Conversion21/1 -> Gain3/1
  Length Conversion8/1 -> Bus Creator1/5  "VelocityZ"
  Data Type Conversion17/1 -> Gain14/1
  Radians to Degrees1/1 -> Bus Creator1/8  "Pitch"
  Length Conversion7/1 -> Bus Creator1/4  "VelocityY"
  Constant3/1 -> Divide2/1
  Gain5/1 -> Length Conversion10/1
  Length Conversion10/1 -> Bus Creator1/11  "AccelerationY"
  Gain7/1 -> Length Conversion11/1
  Radians to Degrees/1 -> Bus Creator1/7  "Roll"
  Divide1/1 -> Sin/1
  Bus Selector1/8 -> Data Type Conversion21/1  "<Pitch>"
  Data Type Conversion10/1 -> Divide2/2
  Data Type Conversion30/1 -> Bus Creator1/16  "INS_Alignment_State"
  Gain10/1 -> Add6/1
  Radians to Degrees3/1 -> Bus Creator1/6  "Azimuth"
  Length Conversion11/1 -> Bus Creator1/12  "AccelerationZ"
  Constant11/1 -> Divide1/1
  Gain16/1 -> Radians to Degrees3/1
  Gain13/1 -> Length Conversion6/1
  Bus Creator1/1 -> INS_data/1
  In_INS/1 -> Bus Selector1/1
  Gain3/1 -> Gain17/1
  Gain4/1 -> Gain1/1
  Gain2/1 -> Gain9/1
  Gain9/1 -> Radians to Degrees/1
  Gain17/1 -> Radians to Degrees1/1
  Gain1/1 -> Radians to Degrees2/1
  Bus Selector1/1 -> Data Type Conversion14/1  "<INSModeWord>"
  Sum/1 -> Bus Creator1/13, Mux/2  "Latitude_INS"
  MATLAB Function1/1(lat_bias) -> Scope2/3, Sum/2
  Sum1/1 -> Mux1/2, Bus Creator1/14  "Longitude_INS"
  MATLAB Function1/2(lon_bias) -> Scope2/4, Sum1/1
  Mux/1 -> Scope1/1
  Mux1/1 -> Scope1/2
  Data Type Conversion27/1 -> Sum/1, Mux/1
  Data Type Conversion28/1 -> Sum1/2, Mux1/1
  WoW/1 -> Scope2/2, MATLAB Function1/1(WoW)
  time/1 -> Scope2/1, MATLAB Function1/2(time)

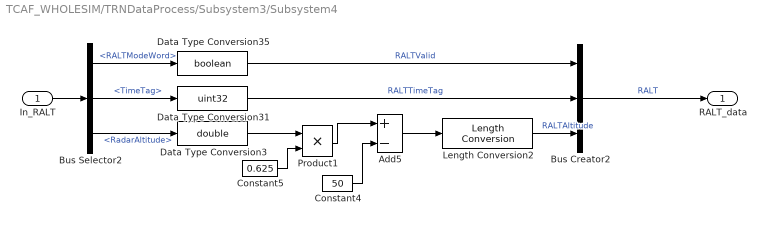
== system TCAF_WHOLESIM/TRNDataProcess/Subsystem3/Subsystem4 ==
  In_RALT : Inport
  Add5 : Sum  Inputs=+-
  Bus Creator2 : BusCreator  Inputs=3  OutDataTypeStr=Bus: TRN_RALT
  Bus Selector2 : BusSelector  OutputSignals=RALTModeWord,TimeTag,RadarAltitude
  Constant4 : Constant  Value=50
  Constant5 : Constant  Value=0.625
  Data Type Conversion3 : DataTypeConversion  OutDataTypeStr=double  SaturateOnIntegerOverflow=off  RndMeth=Floor
  Data Type Conversion31 : DataTypeConversion  OutDataTypeStr=uint32  SaturateOnIntegerOverflow=off  RndMeth=Floor
  Data Type Conversion35 : DataTypeConversion  OutDataTypeStr=boolean  SaturateOnIntegerOverflow=off  RndMeth=Floor
  Length Conversion2 : aerolibconvert2/Length Conversion  IU=ft  OU=m
  Product1 : Product
  RALT_data : Outport
  wires:
  Length Conversion2/1 -> Bus Creator2/3  "RALTAltitude"
  Constant4/1 -> Add5/2
  Bus Creator2/1 -> RALT_data/1  "RALT"
  In_RALT/1 -> Bus Selector2/1
  Data Type Conversion35/1 -> Bus Creator2/1  "RALTValid"
  Add5/1 -> Length Conversion2/1
  Bus Selector2/3 -> Data Type Conversion3/1  "<RadarAltitude>"
  Data Type Conversion3/1 -> Product1/1
  Product1/1 -> Add5/1
  Constant5/1 -> Product1/2
  Data Type Conversion31/1 -> Bus Creator2/2  "RALTTimeTag"
  Bus Selector2/2 -> Data Type Conversion31/1  "<TimeTag>"
  Bus Selector2/1 -> Data Type Conversion35/1  "<RALTModeWord>"

== matlab function TCAF_WHOLESIM/InitNUpdateMapCache/UpdateCache/UpdateCache ==
  data: result output; lat input; lon input; hDEM output
function [result, hDEM] = UpdateCache(lat, lon)
%UpdateCache

% Persistent variables
persistent latPrev lonPrev
if isempty(latPrev)
    latPrev = 0.0;
end
if isempty(lonPrev)
    lonPrev = 0.0;
end

hDEM = 0.0;

% Initialize output
result = int32(1);

if ( abs(lat - latPrev) > 0.05 ) || ( abs(lon - lonPrev) > 0.05)
    result = coder.ceval('UpdateCache', lat, lon);
    hDEM = coder.ceval('MAPGetTerrainHeight', lat, lon);

    if result == 0
        latPrev = lat;
        lonPrev = lon;
    end
else
    
end

== matlab function TCAF_WHOLESIM/InitNUpdateMapCache/InitializeMAP ==
  data: successDTED output; successDVOF output
function [successDTED, successDVOF] = InitializeMAP()
%InitializeMAP

% Persistent variable
persistent firstRun
if isempty(firstRun)
    firstRun = true;
end

% Initialize output
flagDTED = int32(1);
flagDVOF = int32(1);
successDTED = int32(1);
successDVOF = int32(1);

if firstRun
    % Path of DTED data
    pathDTED = 'C:\Users\ASCL\Documents\GitHub\DTNS\MAP\MAP_DB';

    % Length of DETD data path
    strLenDTED = int32(strlength(pathDTED));
    
    % Call [ InitialMap ] : 맵 폴더 위치 설정
    flagDTED = coder.ceval('InitialMap', pathDTED, strLenDTED );
    
    successDTED = flagDTED;

    if (~successDTED)
        firstRun = false;
    end
else
    successDTED = int32(0);
    successDVOF = int32(0);
end

== matlab function TCAF_WHOLESIM/MATFunction_VisualizeWCP ==
  data: wtp input; predictedTraj input; pathDTF input; msd input; pathGCAWS input
function Visualize(wtp, predictedTraj, pathDTF, msd, pathGCAWS)
%VISUALIZE
% 
persistent fHandle subPlot1 subPlot2 tSpanWCP tSpanPT count map ARCSEC2DEG mapSurf predBound yAxisMax

acXY = zeros(2,27);
heading = 0;

% Initialize Figure Handle
if isempty(fHandle)
    fHandle = figure('WindowStyle', 'docked');
end

% Divide and Initailize the Figure
if isempty(subPlot1)
    set(0, 'CurrentFigure', fHandle);
    subPlot1 = subplot(1, 4, 1:2);
    axis equal;
    colormap(fliplr(hsv));
    view(0, 90);
    set(gca, 'Color', [0.3, 0.3, 0.3]);
    xlabel('Longitude [deg]');
    ylabel('Latitude [deg]');
    hold off;
end

% Divide and Initailize the Figure
if isempty(subPlot2)
    subPlot2 = subplot(1, 4, 3:4);
    hold on;
    grid minor;
    xlabel('Time [sec]');
    ylabel('Height [m]');
    axis([-0.5, 20, 0, 2000]);
    hold off;
end

% Initialize tSpanWCP
if isempty(tSpanWCP)
    tSpanWCP = 0:0.5:((length(wtp)-1)*0.5);
end

% Initialize tSpanPT
if isempty(tSpanPT)
    tSpanPT = 0:0.25:((size(predictedTraj, 1)-1)*0.25);
end

% Initialize count
if isempty(count)
    count = 0;    
end

% Initialize yAxisMax
if isempty(yAxisMax) 
    yAxisMax = 2000;
end
% Initialize ARCSEC2DEG
if isempty(ARCSEC2DEG)
    ARCSEC2DEG = (0.000277777777777777);
end

% Initialize map
if isempty(map)
    map = ones(150, 150, 3);

    % Current A/C Position
    latTrue = predictedTraj(1, 1, 1);
    lonTrue = predictedTraj(1, 1, 2);
    
    % Flooring to neighboring Map Grid
    latTrun = floor(latTrue/(3*ARCSEC2DEG)) * (3*ARCSEC2DEG);
    lonTrun = floor(lonTrue/(3*ARCSEC2DEG)) * (3*ARCSEC2DEG);
    
    mapSizeLat = size(map, 1);
    mapSizeLon = size(map, 2);
    % Update map data
    for ii = 1:size(map, 1)
    
        for jj = 1:size(map, 2)
            
            map(ii, jj, 1) = latTrun + (9*ARCSEC2DEG) * ((size(map, 1) - floor(mapSizeLat * 1.5)) + ii);
            map(ii, jj, 2) = lonTrun + (9*ARCSEC2DEG) * ((size(map, 2) - floor(mapSizeLon * 1.5)) + jj);
            
            map(ii, jj, 3) = ...
            coder.ceval('MAPGetTerrainHeight', map(ii, jj, 1), map(ii, jj, 2)); 

            if (ii == size(map, 1)) && (jj == size(map, 2))
                map(ii, jj, 3) = 2200;
            end
            
        end
    
    end
    
end

% Initialize mapSurf: mapSurf plot handle
if isempty(mapSurf)
    set(0, 'CurrentFigure', fHandle);
    subplot(subPlot1);
    hold on;
    mapSurf = surf(map(:,:,2), map(:,:,1), map(:,:,3), 'FaceAlpha', 0.75);
    drawnow;
    hold off;
end

% Initialize predBound: predBound plot handle
if isempty(predBound)
    set(0, 'CurrentFigure', fHandle);
    subplot(subPlot1);
    hold on;
    predBound = plot3([predictedTraj(:,2,2); flipud(predictedTraj(:,3,2))], ...
        [predictedTraj(:,2,1); flipud(predictedTraj(:,3,1))], ...
        [predictedTraj(:,2,3); flipud(predictedTraj(:,3,3))], '-m', 'LineWidth', 3);
    hold off;
end


%%

% Limit & Reset count
if (count >= 800)
    count = 0;
end

% 0.5Hz Event
if rem(count, 200) == 0
    set(0, 'CurrentFigure', fHandle);
    subplot(subPlot1);
    hold on;
    
    % Current A/C Position
    latTrue = predictedTraj(1, 1, 1);
    lonTrue = predictedTraj(1, 1, 2);
    
    % Flooring to neighboring Map Grid
    latTrun = floor(latTrue/(3*ARCSEC2DEG)) * (3*ARCSEC2DEG);
    lonTrun = floor(lonTrue/(3*ARCSEC2DEG)) * (3*ARCSEC2DEG);
    
    mapSizeLat = size(map, 1);
    mapSizeLon = size(map, 2);
    if abs(latTrun-(map(1, 1, 1)+map(end, 1, 1))/2) >= 100*(3*ARCSEC2DEG) || abs(lonTrun-(map(1, 1, 2)+map(1, end, 2))/2) >= 100*(3*ARCSEC2DEG)
        % Update map data
        for ii = 1:size(map, 1)
            for jj = 1:size(map, 2)
                map(ii, jj, 1) = latTrun + (9*ARCSEC2DEG) * ((size(map, 1) - floor(mapSizeLat * 1.5)) + ii);
                map(ii, jj, 2) = lonTrun + (9*ARCSEC2DEG) * ((size(map, 2) - floor(mapSizeLon * 1.5)) + jj);
                map(ii, jj, 3) = ...
                coder.ceval('MAPGetTerrainHeight', map(ii, jj, 1), map(ii, jj, 2)); 
            end
        end
        
        set(mapSurf, 'XData', map(:,:,2), 'YData', map(:,:,1), 'ZData', map(:,:,3));
        drawnow;
    end
    
    % Draw Map
    axis([lonTrun - (3*ARCSEC2DEG)*60, lonTrun + (3*ARCSEC2DEG)*60, latTrun - (3*ARCSEC2DEG)*60, latTrun + (3*ARCSEC2DEG)*60]);
    drawnow;
    hold off;
    
end

% 2.5Hz Event
if rem(count, 40) == 0
    set(0, 'CurrentFigure', fHandle);
    subplot(subPlot1);
    
    hold on;
    latTrue = predictedTraj(1, 1, 1);
    lonTrue = predictedTraj(1, 1, 2);
    heading = getHeadingFromVector([latTrue, lonTrue], [predictedTraj(81, 1, 1), predictedTraj(81, 1, 2)]);
    acXY = drawAircraft( [lonTrue;latTrue], 4.5*ARCSEC2DEG, heading);
    plot3(acXY(1,:), acXY(2,:), predictedTraj(1, 1, 3)*ones(size(acXY(1,:))), '-r')
    
    set(predBound, 'XData', [predictedTraj(:,2,2); flipud(predictedTraj(:,3,2))], ...
    'YData', [predictedTraj(:,2,1); flipud(predictedTraj(:,3,1))], ...
    'ZData', [predictedTraj(:,2,3); flipud(predictedTraj(:,3,3))]);
    
    hold off;
    
    set(0, 'CurrentFigure', fHandle);
    subplot(subPlot2);
    
    nominalTerrain = zeros(size(predictedTraj, 1), 1);
    for nn = 1:size(predictedTraj(:,1,3), 1)
        nominalTerrain(nn) = coder.ceval('MAPGetTerrainHeight', predictedTraj(nn, 1, 1), predictedTraj(nn, 1, 2)); 
%         if nn == 1
%             fprintf("Nominal Terrain(1) - Lat:%f, Lon:%f, Height: %f", predictedTraj(nn, 1, 1), predictedTraj(nn, 1, 2), nominalTerrain(nn));
%         elseif nn == 41
%             fprintf("Nominal Terrain(41) - Lat:%f, Lon:%f, Height: %f", predictedTraj(nn, 1, 1), predictedTraj(nn, 1, 2), nominalTerrain(nn));
%         end
    end
    
    hold on;
    cla
    plot(tSpanPT, nominalTerrain, '-g', 'LineWidth', 5, 'DisplayName', 'Nominal Terrain');
    plot(tSpanWCP, wtp, '-b', 'LineWidth', 5, 'DisplayName', 'WTP');
    plot(tSpanWCP, wtp+msd, '--y', 'LineWidth', 5, 'DisplayName', 'WTP + MSD');
    plot(tSpanPT, predictedTraj(:, 1, 3), '--k', 'LineWidth', 2, 'DisplayName', 'Predicted Nominal Trajectory');
    plot(0, predictedTraj(1, 1, 3), 'ro', 'MarkerSize', 10, 'DisplayName', 'A/C');
    plot(0:0.5:20, pathDTF, '-y', 'DisplayName','DBTF Reference Trajectory', 'LineWidth', 2);
    
    for ii = 1:12
       plot(0:0.5:20, pathGCAWS(:,ii,3));
       
    end
    
    if (predictedTraj(1, 1, 3) > yAxisMax-300)
        axis([-0.5, 20, 0, predictedTraj(1, 1, 3) + 500]);
    elseif (predictedTraj(1, 1, 3) < 1800)
        axis([-0.5, 20, 0, 2000])
    end
    % axis([-1, 20, 300, 800]);
    drawnow;
    hold off; 
    
end

% Update count
count = count + 1;

end


function [acXY] = drawAircraft(centerXY, longLength, heading)
%DRAWAircraft
    % centerXY      (2x1)
    % longLength    (1) [deg]
    % heading       (1) [deg]
    
    acXY = zeros(2, 27);
    translate = ones(2, 27);
    translate(1,:) = translate(1,:) * centerXY(1); 
    translate(2,:) = translate(2,:) * centerXY(2); 
    
    refXY = [ 0, -2, -4, -6,-16,-16,-17,-17, -4, -4, -9,-10, -4,  0,  4, 10,  9,  4,  4, 17, 17, 16, 16,  6,  4,  2,  0;...
             25, 20,  8,  0, -7, -4, -4,-14,-14,-18,-23,-26,-25,-25,-25,-26,-23,-18,-14,-14, -4, -4, -7,  0,  8, 20, 25];
    
    acXY = refXY / 50 * longLength;
    
    rot = [cosd(-heading), -sind(-heading); sind(-heading), cosd(-heading)];
    
    acXY = rot * acXY + translate;
    
end

function [heading] = getHeadingFromVector(fromLatLon, toLatLon)
%GETHEADINGFROMVECTOR
    % fromLatLon (2x1) [deg]
    % toLatLon (2x1) [deg]
    
    dLon = toLatLon(2) - fromLatLon(2);
    
    y = sind(dLon) * cosd(toLatLon(1));
    x = cosd(fromLatLon(1)) * sind(toLatLon(1)) ...
        - sind(fromLatLon(1)) * cosd(toLatLon(1)) * cosd(dLon);
    
    heading = atan2d(y, x);
    heading = rem( heading + 360, 360);

end

== matlab function TCAF_WHOLESIM/ControlFlightCmd ==
  data: inBus input Bus: BUS_FLCC_FLIGHT_CMD; outBus output Bus: BUS_FLCC_FLIGHT_CMD; state input
function outBus = ControlFlightCmd(inBus, state)
%ControlFlightCmd
persistent time dt wayPoint
if isempty(time)
    time = 0.0;
end
if isempty(dt)
    dt = 0.01;
end
if isempty(wayPoint)
    wayPoint = 0;
end

ACTIVATED = true;

% -switchGCAS
SWICH_GCAS_NOT_SELECTED = uint8(0);
SWICH_GCAS_SELECTED     = uint8(1);
SWICH_GCAS_AUTO_GCAS    = uint8(2);

% -switchTF
SWICH_TF_NOT_SELECTED   = uint8(0);
SWICH_TF_SELECTED       = uint8(1);
SWICH_TF_AUTO_TF        = uint8(2);

% -switchRoll
SWITCH_ROLL_ATT_HOLD    = uint8(0);
SWITCH_ROLL_STRG_SEL    = uint8(1);
SWITCH_ROLL_HDG_SEL     = uint8(2);

% -switchPitch
SWITCH_PITCH_AP_OFF     = uint8(0);
SWITCH_PITCH_ATT_HOLD   = uint8(1);
SWITCH_PITCH_ALT_HOLD   = uint8(2);

% Copy
outBus = inBus;

if ACTIVATED
    
    % [Roll] Switch
%     outBus.switchRoll = SWITCH_ROLL_ATT_HOLD;
%     outBus.switchRoll = SWITCH_ROLL_STRG_SEL;
    outBus.switchRoll = SWITCH_ROLL_HDG_SEL;

    % [Pitch] Switch
%     outBus.switchPitch = SWITCH_PITCH_AP_OFF;
%     outBus.switchPitch = SWITCH_PITCH_ATT_HOLD;
    outBus.switchPitch = SWITCH_PITCH_ALT_HOLD;

    % [TF] Switch
%     outBus.switchTF = SWICH_TF_NOT_SELECTED;
    outBus.switchTF = SWICH_TF_SELECTED;
%     outBus.switchTF = SWICH_TF_AUTO_TF;

    % [GCAWS] Switch
%     outBus.switchGCAS = SWICH_GCAS_NOT_SELECTED;
%     outBus.switchGCAS = SWICH_GCAS_SELECTED;
    outBus.switchGCAS = SWICH_GCAS_AUTO_GCAS;

    % [WTPG] Sim: Roll
    %     outBus = SET_ATF(outBus, false, time, 0, inf);
    %     outBus = SET_ROLL_ATT(outBus, 30, time, 20, 20);
    %     outBus = SET_ROLL_ATT(outBus, -30, time, 40, 20);
    %     outBus = SET_ROLL_ATT(outBus, 0, time, 60, inf);

    % [DTF & GCAWS] Feasibility Sim
%     outBus.switchTF = SWICH_TF_SELECTED;
%     outBus.switchGCAS = SWICH_GCAS_AUTO_GCAS;
%     outBus.switchRoll = SWITCH_ROLL_ATT_HOLD;
    %     outBus.switchRoll = uint8(0);
    %     outBus.switchPitch = uint8(2);
    %     outBus.refSpeed = SET_VALUE(outBus.refSpeed, 100, time, 0, 40);
    %     outBus.refSpeed = SET_VALUE(outBus.refSpeed, 100, time, 40, 40);

        outBus.nextAlt = 800;
        outBus.refSpeed = 200;
        outBus.switchRoll = SWITCH_ROLL_HDG_SEL;
        outBus.setHeading = 180;

    switch wayPoint
        case 0
            outBus.nextLat = 35.2;
            outBus.nextLon = 128;
        case 1
            outBus.nextLat = 34.8;
            outBus.nextLon = 128.4;
        case 2
            outBus.nextLat = 35.2;
            outBus.nextLon = 128.8;
        case 3
            outBus.nextLat = 37.0;
            outBus.nextLon = 129;
        otherwise
            outBus.nextLat = 37.0;
            outBus.nextLon = 129;
            outBus.nextAlt = 1000;
    end

    if ( abs(state.latitude - outBus.nextLat) < 0.001 ) && ( abs(state.longitude - outBus.nextLon) < 0.001 )
        wayPoint = wayPoint + 1;
    end

    %     outBus.nextAlt = 800.0;

end

% Update Time
time = time + dt;
end

function out = SET_ATF(in, isATF, curTime, triggerTime, duration)
% -switchTF
SWICH_TF_NOT_SELECTED   = uint8(0);
SWICH_TF_SELECTED       = uint8(1);
SWICH_TF_AUTO_TF        = uint8(2);

out = in;
if (triggerTime <= curTime) && (curTime <= triggerTime+duration)
    if isATF
        out.switchTF = SWICH_TF_AUTO_TF;
    else
        out.switchTF = SWICH_TF_SELECTED;
    end

else
end
end

function out = SET_ROLL_ATT(in, rollAngle, curTime, triggerTime, duration)
% -switchRoll
SWITCH_ROLL_ATT_HOLD    = uint8(0);
SWITCH_ROLL_STRG_SEL    = uint8(1);
SWITCH_ROLL_HDG_SEL     = uint8(2);

out = in;
if (triggerTime <= curTime) && (curTime <= triggerTime+duration)
    out.switchRoll = SWITCH_ROLL_ATT_HOLD;
    out.setRoll = rollAngle;
else
end
end

function out = SET_VALUE(in, value, curTime, triggerTime, duration)
out = in;
if (triggerTime <= curTime) && (curTime <= triggerTime+duration)
    out = value;
else
end
end
